simulink model "baseline_control"  (Simulink 8.4)
settings: Solver=FixedStepDiscrete  StartTime=0.0  StopTime=20.0  FixedStep=SampleTime  RelTol=1e-3
libraries: simulink x1, Controller_Lib x1
settings Model: Creator=austinmurch  LastModifiedBy=brtaylor
settings OptimizationCC: InlineParams=on  SimCompilerOptimization=On
settings HardwareCC: ProdLargestAtomicInteger=Long  ProdLargestAtomicFloat=Double  ProdIntDivRoundTo=Zero  ProdEndianess=BigEndian  ProdHWDeviceType=Freescale->32-bit PowerPC
settings RTWCC: GenCodeOnly=on  GenerateMakefile=off  CustomSourceCode="#include \"../../../Software/FlightCode/control/rtw_grt_control.c\""

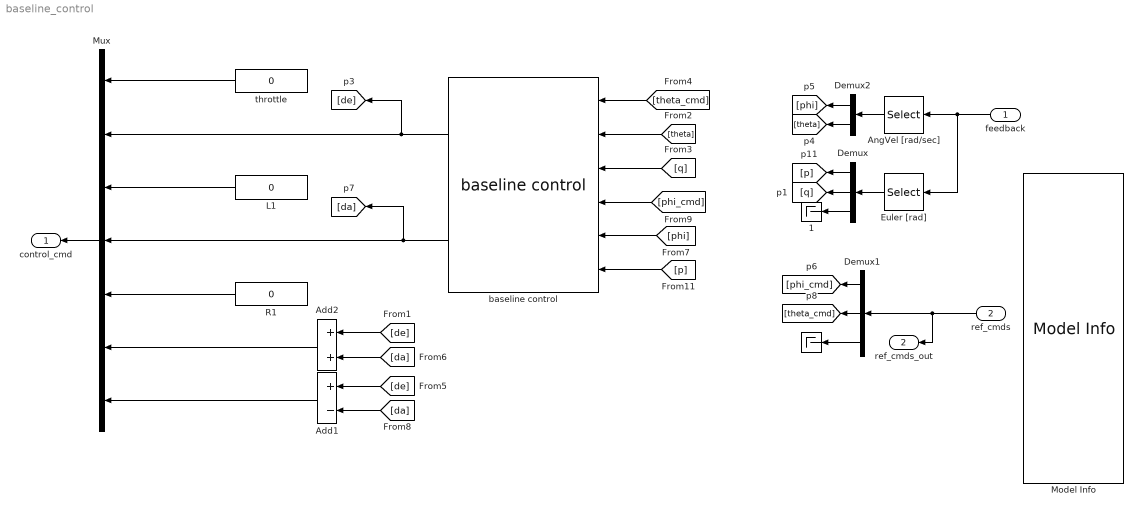
== system baseline_control ==
  feedback : Inport
  ref_cmds : Inport  Port=2
  " " : Terminator
  " 1" : Terminator
  Add1 : Sum  Inputs=+-
  Add2 : Sum
  AngVel [rad/sec] : Selector  InputPortWidth=19  Indices=[1:2]
  Demux : Demux  Outputs=3
  Demux1 : Demux  Outputs=[1 1 10]
  Demux2 : Demux  Outputs=2
  Euler [rad] : Selector  InputPortWidth=19  Indices=[4:6]
  L1 : Constant  Value=0
  Model Info : simulink/Model-Wide Utilities/Model Info  BlockCM=None  Frame=on  DisplayStringWithTags=|  HorizontalTextAlignment=Center  LeftAlignmentValue=0.5  SourceBlockDiagram=baseline_control  TagMaxNumber=20
      | Ref Cmd Port Info
      | 
      | 1. phi_cmd
      | 2. theta_cmd
      | 3. psi_cmd
      | 4. p_cmd
      | 5. q_cmd
      | 6. r_cmd
      | 7. V_s_cmd
      | 8. h_cmd
      | 9. gndtrk_cmd
      | 10. aoa_cmd
      | 11. aos_cmd
      | 12. gamma_cmd
      | 13. signal_0
      | 14. signal_1
      | 15. signal_2
      | 16. signal_3
      | 17. signal_4
      | 18. signal_5
      | 19. signal_6
      | 20. signal_7
      | 21. signal_8
      | 22. signal_9
  Mux : Mux  Inputs=7
  R1 : Constant  Value=0
  baseline control : Controller_Lib/baseline control  pitch=pitch_gains  roll=roll_gains
  throttle : Constant  Value=0
  control_cmd : Outport
  ref_cmds_out : Outport  Port=2
  wires:
  Demux/1 -> [p]
  Demux/2 -> [q]
  Demux/3 -> " 1"/1
  feedback/1 -> AngVel [rad/sec]/1, Euler [rad]/1
  Demux2/2 -> [theta]
  Demux2/1 -> [phi]
  Demux1/1 -> [phi_cmd]
  Demux1/2 -> [theta_cmd]
  Demux1/3 -> " "/1
  Mux/1 -> control_cmd/1
  throttle/1 -> Mux/1
  Euler [rad]/1 -> Demux/1
  AngVel [rad/sec]/1 -> Demux2/1
  ref_cmds/1 -> Demux1/1, ref_cmds_out/1
  [q] -> baseline control/3
  [theta] -> baseline control/2
  [theta_cmd] -> baseline control/1
  [p] -> baseline control/6
  baseline control/1 -> [de], Mux/2
  L1/1 -> Mux/3
  [phi_cmd] -> baseline control/4
  [phi] -> baseline control/5
  R1/1 -> Mux/5
  Add2/1 -> Mux/6
  Add1/1 -> Mux/7
  [de] -> Add2/1
  [de] -> Add1/1
  [da] -> Add2/2
  [da] -> Add1/2
  baseline control/2 -> [da], Mux/4
